simulink model "demodaqsl_aiao_test"  (R2018b)
settings: Solver=FixedStepDiscrete  StartTime=0.0  StopTime=inf  RelTol=1e-3  EnableMultiTasking=on
undefined symbols (not defined in the file): daq
libraries: daqlib x2, dsparch4 x1
settings Model: Creator=The MathWorks, Inc.  LastModifiedBy=79301
settings DataIOCC: LimitDataPoints=on  MaxDataPoints=10000  SaveFormat=Array
settings OptimizationCC: InitFltsAndDblsToZero=on  LifeSpan=inf
settings DebuggingCC: SaveWithParameterizedLinksMsg=none  UnderspecifiedInitializationDetection=Classic  MergeDetectMultiDrivingBlocksExec=none  SignalResolutionControl=TryResolveAllWithWarning  SolverPrmCheckMsg=warning  FcnCallInpInsideContextMsg=warning  LibraryContextMissingDiagnostic=none  SFUnexpectedBacktrackingDiag=warning  SFNoUnconditionalDefaultTransitionDiag=warning  SFExecutionAtInitializationDiag=none
settings HardwareCC: ProdBitPerPointer=32  ProdBitPerSizeT=32  ProdBitPerPtrDiffT=32  ProdLargestAtomicFloat=None  ProdIntDivRoundTo=Undefined  ProdEndianess=Unspecified  ProdWordSize=32  ProdHWDeviceType=32-bit Generic
settings ModelReferenceCC: PropagateSignalLabelsOutOfModel=off
settings SFSimCC: SimUseLocalCustomCode=off
settings RTWCC: RTWUseLocalCustomCode=off
settings CodeAppCC: StateflowObjectComments=on
settings GRTTargetCC: TargetFcnLib=ansi_tfl_tmw.mat  TargetLangStandard=C89/C90 (ANSI)  CombineOutputUpdateFcns=off  GRTInterface=on
settings ConfigComp: CovMetricSettings=dw  CovHtmlReporting=on  CovSaveCumulativeToWorkspaceVar=on  CovSaveSingleToWorkspaceVar=on  CovShowResultsExplorer=off  CovExternalEMLEnable=off

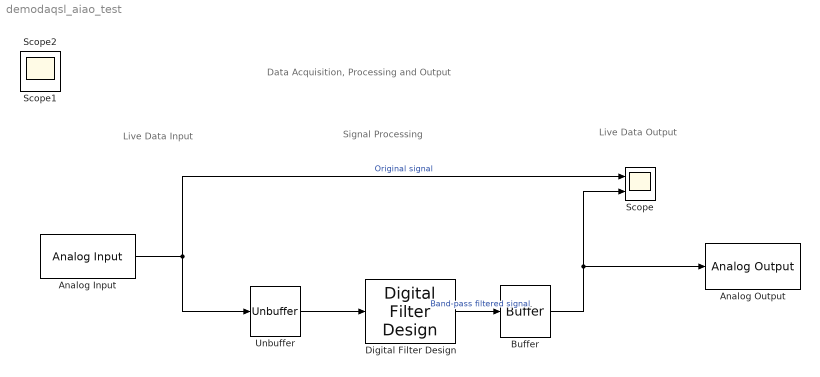
== system demodaqsl_aiao_test ==
  note: Live Data Input
  note: Signal Processing
  note: Live Data Output
  note: Data Acquisition, Processing and Output
  Analog Input : daqlib/Analog Input  DeviceMenu=ni myDAQ1 (NI myDAQ)  Device=ni myDAQ1 (NI myDAQ)  ObjConstructor=daq.createSession('ni')  NChannelsSelected=1  Channels=1$ai0$$myDAQ1$1$2$1$1$#0$ai1$$myDAQ1$1$2$1$1$#  NPorts=1 for all channels  SampleRate=8000  ActualRate=8000  ScansPerTrigger=1600  OutputTimestamp=off  AcqMode=1  NumFrameBuffer=100  OutputTriggertime=off
      settings: SourceProductName=Data Acquisition Toolbox  SourceProductBaseCode=DA
  Analog Output : daqlib/Analog Output  DeviceMenu=ni myDAQ1 (NI myDAQ)  Device=ni myDAQ1 (NI myDAQ)  ObjConstructor=daq.createSession('ni')  NChannelsSelected=1  Channels=1$ao0$$myDAQ1$1$2$N/A$#0$ao1$$myDAQ1$1$2$N/A$#  NPorts=1 for all channels  SampleRate=8000  ActualRate=8000
      settings: SourceProductName=Data Acquisition Toolbox  SourceProductBaseCode=DA
  Buffer : Buffer  N=1600  OutputFrames=off
  Digital Filter Design : dsparch4/Digital Filter Design  mwdsp_browser_bugfix_var=off
  Scope : Scope  NumInputPorts=2
  Unbuffer : Unbuffer
  Scope1 : Scope
  Scope2 : Scope
  wires:
  Digital Filter Design/1 -> Buffer/1  "Band-pass filtered signal"
  Analog Input/1 -> Unbuffer/1, Scope/1  "Original signal"
  Unbuffer/1 -> Digital Filter Design/1
  Buffer/1 -> Scope/2, Analog Output/1
